simulink library "monroe_library"  (R2012b)
settings: Solver=ode45  StartTime=0.0  StopTime=10.0  RelTol=1e-3
values from neighbouring files (symbols this model uses):
  input_bit_width = ', num2str(input_bit_width))    [fft_direct_draw.m]
undefined symbols (not defined in the file or in its folder): gcbh, xlBlockLoadCallback
libraries: xbsIndex_r4 x1880, monroe_library x159, casper_library x13, xps_library x1
(part 5 of 43)

== system monroe_library/direct_coeff_gen ==
  sync : Inport
  bulk_delay_1 : Subsystem
  bulk_delay_2 : Subsystem
  bulk_delay_3 : Subsystem
  coeff_gen_stage_1_group_1 : Subsystem
  coeff_gen_stage_1_group_2 : Subsystem
  coeff_gen_stage_1_group_3 : Subsystem
  coeff_gen_stage_1_group_4 : Subsystem
  coeff_gen_stage_2_group_1 : Subsystem
  coeff_gen_stage_2_group_2 : Subsystem
  coeff_gen_stage_2_group_3 : Subsystem
  coeff_gen_stage_2_group_4 : Subsystem
  coeff_gen_stage_3_group_1 : Subsystem
  coeff_gen_stage_3_group_2 : Subsystem
  coeff_gen_stage_3_group_3 : Subsystem
  coeff_gen_stage_3_group_4 : Subsystem
  concat_stage_1 : xbsIndex_r4/Concat  num_inputs=4  dbl_ovrd=off  block_type=concat
  concat_stage_2 : xbsIndex_r4/Concat  num_inputs=4  dbl_ovrd=off  block_type=concat
  concat_stage_3 : xbsIndex_r4/Concat  num_inputs=4  dbl_ovrd=off  block_type=concat
  delay_sync_{1..2,4..5} (4 alike) : xbsIndex_r4/Delay  en=off  latency=1  dbl_ovrd=off  reg_retiming=off  block_type=delay
  delay_sync_3 : xbsIndex_r4/Delay  en=off  latency=36  dbl_ovrd=off  reg_retiming=off  block_type=delay
  coeff_stg1 : Outport
  coeff_stg2 : Outport  Port=2
  coeff_stg3 : Outport  Port=3
  sync_out : Outport  Port=4
  wires:
  sync/1 -> delay_sync_1/1, bulk_delay_1/4(in4), bulk_delay_1/3(in3), bulk_delay_1/2(in2), bulk_delay_1/1(in1)
  bulk_delay_1/1(out1) -> bulk_delay_2/1(in1), coeff_gen_stage_1_group_1/1(sync)
  bulk_delay_1/2(out2) -> bulk_delay_2/2(in2), coeff_gen_stage_1_group_2/1(sync)
  bulk_delay_1/3(out3) -> bulk_delay_2/3(in3), coeff_gen_stage_1_group_3/1(sync)
  bulk_delay_1/4(out4) -> bulk_delay_2/4(in4), coeff_gen_stage_1_group_4/1(sync)
  bulk_delay_2/1(out1) -> bulk_delay_3/1(in1), coeff_gen_stage_2_group_1/1(sync)
  bulk_delay_2/2(out2) -> bulk_delay_3/2(in2), coeff_gen_stage_2_group_2/1(sync)
  bulk_delay_2/3(out3) -> bulk_delay_3/3(in3), coeff_gen_stage_2_group_3/1(sync)
  bulk_delay_2/4(out4) -> bulk_delay_3/4(in4), coeff_gen_stage_2_group_4/1(sync)
  delay_sync_5/1 -> sync_out/1
  delay_sync_4/1 -> delay_sync_5/1
  delay_sync_3/1 -> delay_sync_4/1
  delay_sync_2/1 -> delay_sync_3/1
  delay_sync_1/1 -> delay_sync_2/1
  concat_stage_3/1 -> coeff_stg3/1
  coeff_gen_stage_3_group_4/1(coeff) -> concat_stage_3/4
  coeff_gen_stage_3_group_3/1(coeff) -> concat_stage_3/3
  coeff_gen_stage_3_group_2/1(coeff) -> concat_stage_3/2
  coeff_gen_stage_3_group_1/1(coeff) -> concat_stage_3/1
  bulk_delay_3/4(out4) -> coeff_gen_stage_3_group_4/1(sync)
  bulk_delay_3/3(out3) -> coeff_gen_stage_3_group_3/1(sync)
  bulk_delay_3/2(out2) -> coeff_gen_stage_3_group_2/1(sync)
  bulk_delay_3/1(out1) -> coeff_gen_stage_3_group_1/1(sync)
  concat_stage_2/1 -> coeff_stg2/1
  coeff_gen_stage_2_group_4/1(coeff) -> concat_stage_2/4
  coeff_gen_stage_2_group_3/1(coeff) -> concat_stage_2/3
  coeff_gen_stage_2_group_2/1(coeff) -> concat_stage_2/2
  coeff_gen_stage_2_group_1/1(coeff) -> concat_stage_2/1
  concat_stage_1/1 -> coeff_stg1/1
  coeff_gen_stage_1_group_4/1(coeff) -> concat_stage_1/4
  coeff_gen_stage_1_group_3/1(coeff) -> concat_stage_1/3
  coeff_gen_stage_1_group_2/1(coeff) -> concat_stage_1/2
  coeff_gen_stage_1_group_1/1(coeff) -> concat_stage_1/1

== system monroe_library/double_delay_bram_external_counter ==
  note: The delay length pramater is used to set the depth of the RAM.
  inA : Inport
  inB : Inport  Port=2
  count : Inport  Port=3
  Concat : xbsIndex_r4/Concat  num_inputs=2  dbl_ovrd=off  block_type=concat
  Concat1 : S-Function  LoadFcn=xlBlockLoadCallback(gcbh);  FunctionName=sysgen  Parameters=ptable_  EnableBusSupport=off  mask(Xilinx Bus Concatenator Block){infoedit=Concatenates two or more inputs.  Output will be cast to an unsigned value with the binary point at zero., num_inputs=2, dbl_ovrd_sgadvanced=, dbl_ovrd=off, has_advanced_control=0, sggui_pos=-1,-1,-1,-1, block_type=concat, block_version=, sg_icon_stat=60,60,2,1,white,blue,0,16398980,right,,[ ],[ ], sg_mask_display=|, sg_list_contents=, sg_blockgui_xml=}
      mask sg_mask_display=|
      | fprintf('','COMMENT: begin icon graphics');
      | patch([0 60 60 0 0 ],[0 0 60 60 0 ],[0.77 0.82 0.91 ]);
      | plot([0 60 60 0 0 ],[0 0 60 60 0 ]);
      | patch([12.2 23.76 31.76 39.76 47.76 31.76 20.2 12.2 ],[38.88 38.88 46.88 38.88 46.88 46.88 46.88 38.88 ],[1 1 1 ]);
      | patch([20.2 31.76 23.76 12.2 20.2 ],[30.88 30.88 38.88 38.88 30.88 ],[0.931 0.946 0.973 ]);
      | patch([12.2 23.76 31.76 20.2 12.2 ],[22.88 22.88 30.88 30.88 22.88 ],[1 1 1 ]);
      | patch([20.2 47.76 39.76 31.76 23.76 12.2 20.2 ],[14.88 14.88 22.88 14.88 22.88 22.88 14.88 ],[0.931 0.946 0.973 ]);
      | fprintf('','COMMENT: end icon graphics');
      | fprintf('','COMMENT: begin icon text');
      | color('black');port_label('input',1,'hi');
      | color('black');port_label('input',2,'lo');
      |
      | color('black');disp('\fontsize{20}\}','texmode','on');
      | fprintf('','COMMENT: end icon text');
      mask prompts: infoedit ""; num_inputs "Number of inputs"; dbl_ovrd_sgadvanced ""; dbl_ovrd "Override with doubles"; has_advanced_control ""; sggui_pos ""; block_type ""; block_version ""; sg_icon_stat ""; sg_mask_display ""; sg_list_contents ""; sg_blockgui_xml ""
      mask help: Concatenates two or more inputs. Output will be cast to an unsigned value with the binary point at zero.
      mask init:
      | try
      |   tmp_gcb = gcb;
      |   tmp_gcbh = gcbh;
      |   if (strcmp('SysGenIndex',get_param(bdroot(tmp_gcbh),'tag')) && ~isempty(regexp(bdroot(tmp_gcb), '^xbs', 'once')))
      |     return;
      |   end;
      |   xlMungeMaskParams;
      |   block_config = 'sysgen_blockset:Concat_config';
      | 
      |   block_type='concat';
      | 
      |   serialized_declarations = '{''num_inputs''=>''Int'',''sim_engine''=>''Int'',''sysgen_root''=>''String'',''block_type''=>''String''}';
      |   xlconcat_init();
      |   ptable_ = xlblockprep(get_param(tmp_gcb, 'MaskWSVariables'));
      |   try
      |     xlBlockMoveCallback(tmp_gcbh);
      |   catch 
      |      clear global xl_updateicon_recursion_guard;
      |   end;
      | catch
      |   global dbgsysgen;
      |   if(~isempty(dbgsysgen) && dbgsysgen)
      |     e = regexprep(lasterr, '\n', '\nError: ');
      |     disp(['Error: While running MaskInit code on block ' tmp_gcb ': ' e]);
      |     error(e);
      |   end
      | end
      settings: CopyFcn=xlBlockMoveCallback(gcbh);  DeleteFcn=xlDestroyGui(gcbh);  ModelCloseFcn=xlDestroyGui(gcbh);  PreSaveFcn=xlBlockPreSaveCallback(gcbh);  PostSaveFcn=xlBlockPostSaveCallback(gcbh);  DestroyFcn=xlDestroyGui(gcbh);  OpenFcn=xlOpenGui(gcbh, 'concat_gui.xml', @xlmagicenablement, -1)  CloseFcn=xlDestroyGui(gcbh);  MoveFcn=xlBlockMoveCallback(gcbh);
      mask Help: eval('');xlDoc('-book','sysgen','-topic','Concat');
      mask Display:
      | fprintf('','COMMENT: begin icon graphics');
      | patch([0 60 60 0 0 ],[0 0 60 60 0 ],[0.77 0.82 0.91 ]);
      | plot([0 60 60 0 0 ],[0 0 60 60 0 ]);
      | patch([12.2 23.76 31.76 39.76 47.76 31.76 20.2 12.2 ],[38.88 38.88 46.88 38.88 46.88 46.88 46.88 38.88 ],[1 1 1 ]);
      | patch([20.2 31.76 23.76 12.2 20.2 ],[30.88 30.88 38.88 38.88 30.88 ],[0.931 0.946 0.973 ]);
      | patch([12.2 23.76 31.76 20.2 12.2 ],[22.88 22.88 30.88 30.88 22.88 ],[1 1 1 ]);
      | patch([20.2 47.76 39.76 31.76 23.76 12.2 20.2 ],[14.88 14.88 22.88 14.88 22.88 22.88 14.88 ],[0.931 0.946 0.973 ]);
      | fprintf('','COMMENT: end icon graphics');
      | fprintf('','COMMENT: begin icon text');
      | color('black');port_label('input',1,'hi');
      | color('black');port_label('input',2,'lo');
      | 
      | color('black');disp('\fontsize{20}\}','texmode','on');
      | fprintf('','COMMENT: end icon text');
  Constant1 : xbsIndex_r4/Constant  arith_type=Boolean  const=1  n_bits=1  bin_pt=0  explicit_period=on  period=1  equ=P=C  opselect=C  inp2=PCIN>>17  opr=+  inp1=P  carry=CIN  dbl_ovrd=off  block_type=constant
      settings: block_version=9.1.01
  Constant2 : xbsIndex_r4/Constant  arith_type=Boolean  const=1  n_bits=1  bin_pt=0  explicit_period=on  period=1  equ=P=C  opselect=C  inp2=PCIN>>17  opr=+  inp1=P  carry=CIN  dbl_ovrd=off  block_type=constant
      settings: block_version=9.1.01
  Constant3 : S-Function  LoadFcn=xlBlockLoadCallback(gcbh);  FunctionName=sysgen  Parameters=ptable_  EnableBusSupport=off  mask(Xilinx Constant Block Block){arith_type_sgadvanced=, arith_type=Boolean, const=0, n_bits=1, bin_pt=0, explicit_period_sgadvanced=, explicit_period=on, period=1, dsp48_infoedit=The use of this block for DSP48 instructions is deprecated.  Please use the Opmode block., equ=P=C, opselect_sgadvanced=, opselect=C, inp2_sgadvanced=, inp2=PCIN>>17, opr_sgadvanced=, opr=+, inp1_sgadvanced=, inp1=P, carry_sgadvanced=, carry=CIN, dbl_ovrd_sgadvanced=, dbl_ovrd=off, has_advanced_control=0, sggui_pos=-1,-1,-1,-1, block_type=constant, block_version=9.1.01, sg_icon_stat=35,24,0,1,white,blue,0,bf4ddd8b,right,,[ ],[ ], sg_mask_display=|, sg_list_contents=, sg_blockgui_xml=}
      mask sg_mask_display=|
      | fprintf('','COMMENT: begin icon graphics');
      | patch([0 35 35 0 0 ],[0 0 24 24 0 ],[0.77 0.82 0.91 ]);
      | plot([0 35 35 0 0 ],[0 0 24 24 0 ]);
      | patch([10.325 14.66 17.66 20.66 23.66 17.66 13.325 10.325 ],[15.33 15.33 18.33 15.33 18.33 18.33 18.33 15.33 ],[1 1 1 ]);
      | patch([13.325 17.66 14.66 10.325 13.325 ],[12.33 12.33 15.33 15.33 12.33 ],[0.931 0.946 0.973 ]);
      | patch([10.325 14.66 17.66 13.325 10.325 ],[9.33 9.33 12.33 12.33 9.33 ],[1 1 1 ]);
      | patch([13.325 23.66 20.66 17.66 14.66 10.325 13.325 ],[6.33 6.33 9.33 6.33 9.33 9.33 6.33 ],[0.931 0.946 0.973 ]);
      | fprintf('','COMMENT: end icon graphics');
      | fprintf('','COMMENT: begin icon text');
      | color('black');port_label('output',1,'0');
      | fprintf('','COMMENT: end icon text');
      mask prompts: arith_type_sgadvanced ""; arith_type "Type"; const "Constant value"; n_bits "Number of bits"; bin_pt "Binary point"; explicit_period_sgadvanced ""; explicit_period "Sampled constant"; period "Sample period"; dsp48_infoedit ""; equ "DSP48 operation"; opselect_sgadvanced ""; opselect "Operation select"; inp2_sgadvanced ""; inp2 "Z mux"; opr_sgadvanced ""; opr "Operand"; inp1_sgadvanced ""; inp1 "YX muxes"; carry_sgadvanced ""; carry "Carry input"; dbl_ovrd_sgadvanced ""; dbl_ovrd "Override with doubles"; has_advanced_control ""; sggui_pos ""; block_type ""; block_version ""; sg_icon_stat ""; sg_mask_display ""; sg_list_contents ""; sg_blockgui_xml ""
      mask help: Xilinx Constant Block
      mask init:
      | try
      |   tmp_gcb = gcb;
      |   tmp_gcbh = gcbh;
      |   if (strcmp('SysGenIndex',get_param(bdroot(tmp_gcbh),'tag')) && ~isempty(regexp(bdroot(tmp_gcb), '^xbs', 'once')))
      |     return;
      |   end;
      |   xlMungeMaskParams;
      |   block_config = 'sysgen_blockset:Constant_config';
      | 
      |   block_type='constant';
      | 
      |   serialized_declarations = '{''arith_type''=>''Int'',''bin_pt''=>''Int'',''carry''=>''Int'',''const''=>''Double'',''dbl_ovrd''=>''Int'',''explicit_period''=>''Int'',''inp1''=>''Int'',''inp2''=>''Int'',''n_bits''=>''Int'',''opr''=>''Int'',''opselect''=>''Int'',''period''=>''Double'',''block_type''=>''String''}';
      |   xlconstant_init();
      |   ptable_ = xlblockprep(get_param(tmp_gcb, 'MaskWSVariables'));
      |   try
      |     xlBlockMoveCallback(tmp_gcbh);
      |   catch 
      |      clear global xl_updateicon_recursion_guard;
      |   end;
      | catch
      |   global dbgsysgen;
      |   if(~isempty(dbgsysgen) && dbgsysgen)
      |     e = regexprep(lasterr, '\n', '\nError: ');
      |     disp(['Error: While running MaskInit code on block ' tmp_gcb ': ' e]);
      |     error(e);
      |   end
      | end
      settings: CopyFcn=xlBlockMoveCallback(gcbh);  DeleteFcn=xlDestroyGui(gcbh);  ModelCloseFcn=xlDestroyGui(gcbh);  PreSaveFcn=xlBlockPreSaveCallback(gcbh);  PostSaveFcn=xlBlockPostSaveCallback(gcbh);  DestroyFcn=xlDestroyGui(gcbh);  OpenFcn=xlOpenGui(gcbh, 'constant_gui.xml', @constantenablement, @constantaction)  CloseFcn=xlDestroyGui(gcbh);  MoveFcn=xlBlockMoveCallback(gcbh);
      mask Help: eval('');xlDoc('-book','sysgen','-topic','Constant');
      mask TypeOptions arith_type: Boolean | Signed (2's comp) | Unsigned | DSP48 Instruction
      mask TypeOptions opselect: C + A*B | PCIN + A*B | P + A*B | A * B | C + A:B | C - A:B | C | Custom
      mask TypeOptions inp2: 0 | PCIN | P | C | PCIN>>17 | P>>17
      mask TypeOptions opr: + | -
      mask TypeOptions inp1: 0 | P | A:B | A*B | C | P+C | A:B+C
      mask TypeOptions carry: 0 | 1 | CIN | ~SIGN(P or PCIN) | ~SIGN(A*B or A:B) | ~SIGND(A*B or A:B)
      mask Display:
      | fprintf('','COMMENT: begin icon graphics');
      | patch([0 35 35 0 0 ],[0 0 24 24 0 ],[0.77 0.82 0.91 ]);
      | plot([0 35 35 0 0 ],[0 0 24 24 0 ]);
      | patch([10.325 14.66 17.66 20.66 23.66 17.66 13.325 10.325 ],[15.33 15.33 18.33 15.33 18.33 18.33 18.33 15.33 ],[1 1 1 ]);
      | patch([13.325 17.66 14.66 10.325 13.325 ],[12.33 12.33 15.33 15.33 12.33 ],[0.931 0.946 0.973 ]);
      | patch([10.325 14.66 17.66 13.325 10.325 ],[9.33 9.33 12.33 12.33 9.33 ],[1 1 1 ]);
      | patch([13.325 23.66 20.66 17.66 14.66 10.325 13.325 ],[6.33 6.33 9.33 6.33 9.33 9.33 6.33 ],[0.931 0.946 0.973 ]);
      | fprintf('','COMMENT: end icon graphics');
      | fprintf('','COMMENT: begin icon text');
      | color('black');port_label('output',1,'0');
      | fprintf('','COMMENT: end icon text');
  Dual Port RAM : xbsIndex_r4/Dual Port RAM  depth=2^ceil(log(2*(delay_len-bram_latency))/log(2))  initVector=0  distributed_mem=Block RAM  init_a=0  init_b=0  rst_a=off  rst_b=off  en_a=off  en_b=off  latency=bram_latency  write_mode_A=Read Before Write  write_mode_B=Read Before Write  dbl_ovrd=off  optimize=Area  use_rpm=on  block_type=dpram
      settings: block_version=11.4
  outA : Outport
  outB : Outport  Port=2
  wires:
  Constant3/1 -> Concat1/1
  Concat1/1 -> Dual Port RAM/4
  Concat/1 -> Dual Port RAM/1
  Constant1/1 -> Concat/1
  count/1 -> Concat1/2, Concat/2
  Constant2/1 -> Dual Port RAM/3, Dual Port RAM/6
  inB/1 -> Dual Port RAM/5
  inA/1 -> Dual Port RAM/2
  Dual Port RAM/2 -> outB/1
  Dual Port RAM/1 -> outA/1

== system monroe_library/double_delay_bram_fast ==
  inA : Inport
  inB : Inport  Port=2
  Concat : xbsIndex_r4/Concat  num_inputs=2  dbl_ovrd=off  block_type=concat
  Concat1 : S-Function  LoadFcn=xlBlockLoadCallback(gcbh);  FunctionName=sysgen  Parameters=ptable_  EnableBusSupport=off  mask(Xilinx Bus Concatenator Block){infoedit=Concatenates two or more inputs.  Output will be cast to an unsigned value with the binary point at zero., num_inputs=2, dbl_ovrd_sgadvanced=, dbl_ovrd=off, has_advanced_control=0, sggui_pos=-1,-1,-1,-1, block_type=concat, block_version=, sg_icon_stat=60,60,2,1,white,blue,0,16398980,right,,[ ],[ ], sg_mask_display=|, sg_list_contents=, sg_blockgui_xml=}
      mask sg_mask_display=|
      | fprintf('','COMMENT: begin icon graphics');
      | patch([0 60 60 0 0 ],[0 0 60 60 0 ],[0.77 0.82 0.91 ]);
      | plot([0 60 60 0 0 ],[0 0 60 60 0 ]);
      | patch([12.2 23.76 31.76 39.76 47.76 31.76 20.2 12.2 ],[38.88 38.88 46.88 38.88 46.88 46.88 46.88 38.88 ],[1 1 1 ]);
      | patch([20.2 31.76 23.76 12.2 20.2 ],[30.88 30.88 38.88 38.88 30.88 ],[0.931 0.946 0.973 ]);
      | patch([12.2 23.76 31.76 20.2 12.2 ],[22.88 22.88 30.88 30.88 22.88 ],[1 1 1 ]);
      | patch([20.2 47.76 39.76 31.76 23.76 12.2 20.2 ],[14.88 14.88 22.88 14.88 22.88 22.88 14.88 ],[0.931 0.946 0.973 ]);
      | fprintf('','COMMENT: end icon graphics');
      | fprintf('','COMMENT: begin icon text');
      | color('black');port_label('input',1,'hi');
      | color('black');port_label('input',2,'lo');
      |
      | color('black');disp('\fontsize{20}\}','texmode','on');
      | fprintf('','COMMENT: end icon text');
      mask prompts: infoedit ""; num_inputs "Number of inputs"; dbl_ovrd_sgadvanced ""; dbl_ovrd "Override with doubles"; has_advanced_control ""; sggui_pos ""; block_type ""; block_version ""; sg_icon_stat ""; sg_mask_display ""; sg_list_contents ""; sg_blockgui_xml ""
      mask help: Concatenates two or more inputs. Output will be cast to an unsigned value with the binary point at zero.
      mask init: same as monroe_library/double_delay_bram_external_counter/Concat1
      settings: CopyFcn=xlBlockMoveCallback(gcbh);  DeleteFcn=xlDestroyGui(gcbh);  ModelCloseFcn=xlDestroyGui(gcbh);  PreSaveFcn=xlBlockPreSaveCallback(gcbh);  PostSaveFcn=xlBlockPostSaveCallback(gcbh);  DestroyFcn=xlDestroyGui(gcbh);  OpenFcn=xlOpenGui(gcbh, 'concat_gui.xml', @xlmagicenablement, -1)  CloseFcn=xlDestroyGui(gcbh);  MoveFcn=xlBlockMoveCallback(gcbh);
      mask Help: eval('');xlDoc('-book','sysgen','-topic','Concat');
      mask Display:
      | fprintf('','COMMENT: begin icon graphics');
      | patch([0 60 60 0 0 ],[0 0 60 60 0 ],[0.77 0.82 0.91 ]);
      | plot([0 60 60 0 0 ],[0 0 60 60 0 ]);
      | patch([12.2 23.76 31.76 39.76 47.76 31.76 20.2 12.2 ],[38.88 38.88 46.88 38.88 46.88 46.88 46.88 38.88 ],[1 1 1 ]);
      | patch([20.2 31.76 23.76 12.2 20.2 ],[30.88 30.88 38.88 38.88 30.88 ],[0.931 0.946 0.973 ]);
      | patch([12.2 23.76 31.76 20.2 12.2 ],[22.88 22.88 30.88 30.88 22.88 ],[1 1 1 ]);
      | patch([20.2 47.76 39.76 31.76 23.76 12.2 20.2 ],[14.88 14.88 22.88 14.88 22.88 22.88 14.88 ],[0.931 0.946 0.973 ]);
      | fprintf('','COMMENT: end icon graphics');
      | fprintf('','COMMENT: begin icon text');
      | color('black');port_label('input',1,'hi');
      | color('black');port_label('input',2,'lo');
      | 
      | color('black');disp('\fontsize{20}\}','texmode','on');
      | fprintf('','COMMENT: end icon text');
  Constant1 : xbsIndex_r4/Constant  arith_type=Boolean  const=1  n_bits=1  bin_pt=0  explicit_period=on  period=1  equ=P=C  opselect=C  inp2=PCIN>>17  opr=+  inp1=P  carry=CIN  dbl_ovrd=off  block_type=constant
      settings: block_version=9.1.01
  Constant2 : xbsIndex_r4/Constant  arith_type=Boolean  const=1  n_bits=1  bin_pt=0  explicit_period=on  period=1  equ=P=C  opselect=C  inp2=PCIN>>17  opr=+  inp1=P  carry=CIN  dbl_ovrd=off  block_type=constant
      settings: block_version=9.1.01
  Constant3 : S-Function  LoadFcn=xlBlockLoadCallback(gcbh);  FunctionName=sysgen  Parameters=ptable_  EnableBusSupport=off  mask(Xilinx Constant Block Block){arith_type_sgadvanced=, arith_type=Boolean, const=0, n_bits=1, bin_pt=0, explicit_period_sgadvanced=, explicit_period=on, period=1, dsp48_infoedit=The use of this block for DSP48 instructions is deprecated.  Please use the Opmode block., equ=P=C, opselect_sgadvanced=, opselect=C, inp2_sgadvanced=, inp2=PCIN>>17, opr_sgadvanced=, opr=+, inp1_sgadvanced=, inp1=P, carry_sgadvanced=, carry=CIN, dbl_ovrd_sgadvanced=, dbl_ovrd=off, has_advanced_control=0, sggui_pos=-1,-1,-1,-1, block_type=constant, block_version=9.1.01, sg_icon_stat=35,24,0,1,white,blue,0,bf4ddd8b,right,,[ ],[ ], sg_mask_display=|, sg_list_contents=, sg_blockgui_xml=}
      mask sg_mask_display=|
      | fprintf('','COMMENT: begin icon graphics');
      | patch([0 35 35 0 0 ],[0 0 24 24 0 ],[0.77 0.82 0.91 ]);
      | plot([0 35 35 0 0 ],[0 0 24 24 0 ]);
      | patch([10.325 14.66 17.66 20.66 23.66 17.66 13.325 10.325 ],[15.33 15.33 18.33 15.33 18.33 18.33 18.33 15.33 ],[1 1 1 ]);
      | patch([13.325 17.66 14.66 10.325 13.325 ],[12.33 12.33 15.33 15.33 12.33 ],[0.931 0.946 0.973 ]);
      | patch([10.325 14.66 17.66 13.325 10.325 ],[9.33 9.33 12.33 12.33 9.33 ],[1 1 1 ]);
      | patch([13.325 23.66 20.66 17.66 14.66 10.325 13.325 ],[6.33 6.33 9.33 6.33 9.33 9.33 6.33 ],[0.931 0.946 0.973 ]);
      | fprintf('','COMMENT: end icon graphics');
      | fprintf('','COMMENT: begin icon text');
      | color('black');port_label('output',1,'0');
      | fprintf('','COMMENT: end icon text');
      mask prompts: arith_type_sgadvanced ""; arith_type "Type"; const "Constant value"; n_bits "Number of bits"; bin_pt "Binary point"; explicit_period_sgadvanced ""; explicit_period "Sampled constant"; period "Sample period"; dsp48_infoedit ""; equ "DSP48 operation"; opselect_sgadvanced ""; opselect "Operation select"; inp2_sgadvanced ""; inp2 "Z mux"; opr_sgadvanced ""; opr "Operand"; inp1_sgadvanced ""; inp1 "YX muxes"; carry_sgadvanced ""; carry "Carry input"; dbl_ovrd_sgadvanced ""; dbl_ovrd "Override with doubles"; has_advanced_control ""; sggui_pos ""; block_type ""; block_version ""; sg_icon_stat ""; sg_mask_display ""; sg_list_contents ""; sg_blockgui_xml ""
      mask help: Xilinx Constant Block
      mask init: same as monroe_library/double_delay_bram_external_counter/Constant3
      settings: CopyFcn=xlBlockMoveCallback(gcbh);  DeleteFcn=xlDestroyGui(gcbh);  ModelCloseFcn=xlDestroyGui(gcbh);  PreSaveFcn=xlBlockPreSaveCallback(gcbh);  PostSaveFcn=xlBlockPostSaveCallback(gcbh);  DestroyFcn=xlDestroyGui(gcbh);  OpenFcn=xlOpenGui(gcbh, 'constant_gui.xml', @constantenablement, @constantaction)  CloseFcn=xlDestroyGui(gcbh);  MoveFcn=xlBlockMoveCallback(gcbh);
      mask Help: eval('');xlDoc('-book','sysgen','-topic','Constant');
      mask TypeOptions arith_type: Boolean | Signed (2's comp) | Unsigned | DSP48 Instruction
      mask TypeOptions opselect: C + A*B | PCIN + A*B | P + A*B | A * B | C + A:B | C - A:B | C | Custom
      mask TypeOptions inp2: 0 | PCIN | P | C | PCIN>>17 | P>>17
      mask TypeOptions opr: + | -
      mask TypeOptions inp1: 0 | P | A:B | A*B | C | P+C | A:B+C
      mask TypeOptions carry: 0 | 1 | CIN | ~SIGN(P or PCIN) | ~SIGN(A*B or A:B) | ~SIGND(A*B or A:B)
      mask Display:
      | fprintf('','COMMENT: begin icon graphics');
      | patch([0 35 35 0 0 ],[0 0 24 24 0 ],[0.77 0.82 0.91 ]);
      | plot([0 35 35 0 0 ],[0 0 24 24 0 ]);
      | patch([10.325 14.66 17.66 20.66 23.66 17.66 13.325 10.325 ],[15.33 15.33 18.33 15.33 18.33 18.33 18.33 15.33 ],[1 1 1 ]);
      | patch([13.325 17.66 14.66 10.325 13.325 ],[12.33 12.33 15.33 15.33 12.33 ],[0.931 0.946 0.973 ]);
      | patch([10.325 14.66 17.66 13.325 10.325 ],[9.33 9.33 12.33 12.33 9.33 ],[1 1 1 ]);
      | patch([13.325 23.66 20.66 17.66 14.66 10.325 13.325 ],[6.33 6.33 9.33 6.33 9.33 9.33 6.33 ],[0.931 0.946 0.973 ]);
      | fprintf('','COMMENT: end icon graphics');
      | fprintf('','COMMENT: begin icon text');
      | color('black');port_label('output',1,'0');
      | fprintf('','COMMENT: end icon text');
  Dual Port RAM : xbsIndex_r4/Dual Port RAM  depth=2^ceil(log(2*(delay_len-bram_latency))/log(2))  initVector=0  distributed_mem=Block RAM  init_a=0  init_b=0  rst_a=off  rst_b=off  en_a=off  en_b=off  latency=bram_latency  write_mode_A=Read Before Write  write_mode_B=Read Before Write  dbl_ovrd=off  optimize=Area  use_rpm=on  block_type=dpram
      settings: block_version=11.4
  counter_limited_fast : monroe_library/counter_limited_fast  SystemSampleTime=-1  bit_width=ceil(log(delay_len-bram_latency)/log(2))  count_to=delay_len-bram_latency-1  register_output=register_counter  cheap_counter=((ceil(log(delay_len-bram_latency)/log(2))) < 8)
  outA : Outport
  outB : Outport  Port=2
  wires:
  Dual Port RAM/1 -> outA/1
  Dual Port RAM/2 -> outB/1
  inA/1 -> Dual Port RAM/2
  inB/1 -> Dual Port RAM/5
  Constant2/1 -> Dual Port RAM/6, Dual Port RAM/3
  counter_limited_fast/1 -> Concat/2, Concat1/2
  Constant1/1 -> Concat/1
  Concat/1 -> Dual Port RAM/1
  Concat1/1 -> Dual Port RAM/4
  Constant3/1 -> Concat1/1

== system monroe_library/double_delay_distrib ==
  inA : Inport
  inB : Inport  Port=2
  Concat : xbsIndex_r4/Concat  num_inputs=2  dbl_ovrd=off  block_type=concat
  Concat1 : S-Function  LoadFcn=xlBlockLoadCallback(gcbh);  FunctionName=sysgen  Parameters=ptable_  EnableBusSupport=off  mask(Xilinx Bus Concatenator Block){infoedit=Concatenates two or more inputs.  Output will be cast to an unsigned value with the binary point at zero., num_inputs=2, dbl_ovrd_sgadvanced=, dbl_ovrd=off, has_advanced_control=0, sggui_pos=-1,-1,-1,-1, block_type=concat, block_version=, sg_icon_stat=60,60,2,1,white,blue,0,16398980,right,,[ ],[ ], sg_mask_display=|, sg_list_contents=, sg_blockgui_xml=}
      mask sg_mask_display=|
      | fprintf('','COMMENT: begin icon graphics');
      | patch([0 60 60 0 0 ],[0 0 60 60 0 ],[0.77 0.82 0.91 ]);
      | plot([0 60 60 0 0 ],[0 0 60 60 0 ]);
      | patch([12.2 23.76 31.76 39.76 47.76 31.76 20.2 12.2 ],[38.88 38.88 46.88 38.88 46.88 46.88 46.88 38.88 ],[1 1 1 ]);
      | patch([20.2 31.76 23.76 12.2 20.2 ],[30.88 30.88 38.88 38.88 30.88 ],[0.931 0.946 0.973 ]);
      | patch([12.2 23.76 31.76 20.2 12.2 ],[22.88 22.88 30.88 30.88 22.88 ],[1 1 1 ]);
      | patch([20.2 47.76 39.76 31.76 23.76 12.2 20.2 ],[14.88 14.88 22.88 14.88 22.88 22.88 14.88 ],[0.931 0.946 0.973 ]);
      | fprintf('','COMMENT: end icon graphics');
      | fprintf('','COMMENT: begin icon text');
      | color('black');port_label('input',1,'hi');
      | color('black');port_label('input',2,'lo');
      |
      | color('black');disp('\fontsize{20}\}','texmode','on');
      | fprintf('','COMMENT: end icon text');
      mask prompts: infoedit ""; num_inputs "Number of inputs"; dbl_ovrd_sgadvanced ""; dbl_ovrd "Override with doubles"; has_advanced_control ""; sggui_pos ""; block_type ""; block_version ""; sg_icon_stat ""; sg_mask_display ""; sg_list_contents ""; sg_blockgui_xml ""
      mask help: Concatenates two or more inputs. Output will be cast to an unsigned value with the binary point at zero.
      mask init: same as monroe_library/double_delay_bram_external_counter/Concat1
      settings: CopyFcn=xlBlockMoveCallback(gcbh);  DeleteFcn=xlDestroyGui(gcbh);  ModelCloseFcn=xlDestroyGui(gcbh);  PreSaveFcn=xlBlockPreSaveCallback(gcbh);  PostSaveFcn=xlBlockPostSaveCallback(gcbh);  DestroyFcn=xlDestroyGui(gcbh);  OpenFcn=xlOpenGui(gcbh, 'concat_gui.xml', @xlmagicenablement, -1)  CloseFcn=xlDestroyGui(gcbh);  MoveFcn=xlBlockMoveCallback(gcbh);
      mask Help: eval('');xlDoc('-book','sysgen','-topic','Concat');
      mask Display:
      | fprintf('','COMMENT: begin icon graphics');
      | patch([0 60 60 0 0 ],[0 0 60 60 0 ],[0.77 0.82 0.91 ]);
      | plot([0 60 60 0 0 ],[0 0 60 60 0 ]);
      | patch([12.2 23.76 31.76 39.76 47.76 31.76 20.2 12.2 ],[38.88 38.88 46.88 38.88 46.88 46.88 46.88 38.88 ],[1 1 1 ]);
      | patch([20.2 31.76 23.76 12.2 20.2 ],[30.88 30.88 38.88 38.88 30.88 ],[0.931 0.946 0.973 ]);
      | patch([12.2 23.76 31.76 20.2 12.2 ],[22.88 22.88 30.88 30.88 22.88 ],[1 1 1 ]);
      | patch([20.2 47.76 39.76 31.76 23.76 12.2 20.2 ],[14.88 14.88 22.88 14.88 22.88 22.88 14.88 ],[0.931 0.946 0.973 ]);
      | fprintf('','COMMENT: end icon graphics');
      | fprintf('','COMMENT: begin icon text');
      | color('black');port_label('input',1,'hi');
      | color('black');port_label('input',2,'lo');
      | 
      | color('black');disp('\fontsize{20}\}','texmode','on');
      | fprintf('','COMMENT: end icon text');
  Constant1 : xbsIndex_r4/Constant  arith_type=Boolean  const=1  n_bits=1  bin_pt=0  explicit_period=on  period=1  equ=P=C  opselect=C  inp2=PCIN>>17  opr=+  inp1=P  carry=CIN  dbl_ovrd=off  block_type=constant
      settings: block_version=9.1.01
  Constant2 : xbsIndex_r4/Constant  arith_type=Boolean  const=1  n_bits=1  bin_pt=0  explicit_period=on  period=1  equ=P=C  opselect=C  inp2=PCIN>>17  opr=+  inp1=P  carry=CIN  dbl_ovrd=off  block_type=constant
      settings: block_version=9.1.01
  Constant3 : S-Function  LoadFcn=xlBlockLoadCallback(gcbh);  FunctionName=sysgen  Parameters=ptable_  EnableBusSupport=off  mask(Xilinx Constant Block Block){arith_type_sgadvanced=, arith_type=Boolean, const=0, n_bits=1, bin_pt=0, explicit_period_sgadvanced=, explicit_period=on, period=1, dsp48_infoedit=The use of this block for DSP48 instructions is deprecated.  Please use the Opmode block., equ=P=C, opselect_sgadvanced=, opselect=C, inp2_sgadvanced=, inp2=PCIN>>17, opr_sgadvanced=, opr=+, inp1_sgadvanced=, inp1=P, carry_sgadvanced=, carry=CIN, dbl_ovrd_sgadvanced=, dbl_ovrd=off, has_advanced_control=0, sggui_pos=-1,-1,-1,-1, block_type=constant, block_version=9.1.01, sg_icon_stat=35,24,0,1,white,blue,0,bf4ddd8b,right,,[ ],[ ], sg_mask_display=|, sg_list_contents=, sg_blockgui_xml=}
      mask sg_mask_display=|
      | fprintf('','COMMENT: begin icon graphics');
      | patch([0 35 35 0 0 ],[0 0 24 24 0 ],[0.77 0.82 0.91 ]);
      | plot([0 35 35 0 0 ],[0 0 24 24 0 ]);
      | patch([10.325 14.66 17.66 20.66 23.66 17.66 13.325 10.325 ],[15.33 15.33 18.33 15.33 18.33 18.33 18.33 15.33 ],[1 1 1 ]);
      | patch([13.325 17.66 14.66 10.325 13.325 ],[12.33 12.33 15.33 15.33 12.33 ],[0.931 0.946 0.973 ]);
      | patch([10.325 14.66 17.66 13.325 10.325 ],[9.33 9.33 12.33 12.33 9.33 ],[1 1 1 ]);
      | patch([13.325 23.66 20.66 17.66 14.66 10.325 13.325 ],[6.33 6.33 9.33 6.33 9.33 9.33 6.33 ],[0.931 0.946 0.973 ]);
      | fprintf('','COMMENT: end icon graphics');
      | fprintf('','COMMENT: begin icon text');
      | color('black');port_label('output',1,'0');
      | fprintf('','COMMENT: end icon text');
      mask prompts: arith_type_sgadvanced ""; arith_type "Type"; const "Constant value"; n_bits "Number of bits"; bin_pt "Binary point"; explicit_period_sgadvanced ""; explicit_period "Sampled constant"; period "Sample period"; dsp48_infoedit ""; equ "DSP48 operation"; opselect_sgadvanced ""; opselect "Operation select"; inp2_sgadvanced ""; inp2 "Z mux"; opr_sgadvanced ""; opr "Operand"; inp1_sgadvanced ""; inp1 "YX muxes"; carry_sgadvanced ""; carry "Carry input"; dbl_ovrd_sgadvanced ""; dbl_ovrd "Override with doubles"; has_advanced_control ""; sggui_pos ""; block_type ""; block_version ""; sg_icon_stat ""; sg_mask_display ""; sg_list_contents ""; sg_blockgui_xml ""
      mask help: Xilinx Constant Block
      mask init: same as monroe_library/double_delay_bram_external_counter/Constant3
      settings: CopyFcn=xlBlockMoveCallback(gcbh);  DeleteFcn=xlDestroyGui(gcbh);  ModelCloseFcn=xlDestroyGui(gcbh);  PreSaveFcn=xlBlockPreSaveCallback(gcbh);  PostSaveFcn=xlBlockPostSaveCallback(gcbh);  DestroyFcn=xlDestroyGui(gcbh);  OpenFcn=xlOpenGui(gcbh, 'constant_gui.xml', @constantenablement, @constantaction)  CloseFcn=xlDestroyGui(gcbh);  MoveFcn=xlBlockMoveCallback(gcbh);
      mask Help: eval('');xlDoc('-book','sysgen','-topic','Constant');
      mask TypeOptions arith_type: Boolean | Signed (2's comp) | Unsigned | DSP48 Instruction
      mask TypeOptions opselect: C + A*B | PCIN + A*B | P + A*B | A * B | C + A:B | C - A:B | C | Custom
      mask TypeOptions inp2: 0 | PCIN | P | C | PCIN>>17 | P>>17
      mask TypeOptions opr: + | -
      mask TypeOptions inp1: 0 | P | A:B | A*B | C | P+C | A:B+C
      mask TypeOptions carry: 0 | 1 | CIN | ~SIGN(P or PCIN) | ~SIGN(A*B or A:B) | ~SIGND(A*B or A:B)
      mask Display:
      | fprintf('','COMMENT: begin icon graphics');
      | patch([0 35 35 0 0 ],[0 0 24 24 0 ],[0.77 0.82 0.91 ]);
      | plot([0 35 35 0 0 ],[0 0 24 24 0 ]);
      | patch([10.325 14.66 17.66 20.66 23.66 17.66 13.325 10.325 ],[15.33 15.33 18.33 15.33 18.33 18.33 18.33 15.33 ],[1 1 1 ]);
      | patch([13.325 17.66 14.66 10.325 13.325 ],[12.33 12.33 15.33 15.33 12.33 ],[0.931 0.946 0.973 ]);
      | patch([10.325 14.66 17.66 13.325 10.325 ],[9.33 9.33 12.33 12.33 9.33 ],[1 1 1 ]);
      | patch([13.325 23.66 20.66 17.66 14.66 10.325 13.325 ],[6.33 6.33 9.33 6.33 9.33 9.33 6.33 ],[0.931 0.946 0.973 ]);
      | fprintf('','COMMENT: end icon graphics');
      | fprintf('','COMMENT: begin icon text');
      | color('black');port_label('output',1,'0');
      | fprintf('','COMMENT: end icon text');
  Counter : S-Function  LoadFcn=xlBlockLoadCallback(gcbh);  FunctionName=sysgen  Parameters=ptable_  EnableBusSupport=off  mask(Xilinx Counter Block){infoedit=Hardware notes: Free running counters are the least expensive in hardware.  A count limited counter is implemented by combining a counter with a comparator., cnt_type_sgadvanced=, cnt_type=Count Limited, cnt_to=delay_len-bram_latency-1, operation_sgadvanced=, operation=Up, start_count=0, cnt_by_val=1, arith_type_sgadvanced=, arith_type=Unsigned, n_bits=ceil(log(delay_len-bram_latency)/log(2)), bin_pt=0, load_pin_sgadvanced=, load_pin=off, rst_sgadvanced=, rst=off, en_sgadvanced=, en=off, explicit_period_sgadvanced=, explicit_period=on, period=1, dbl_ovrd_sgadvanced=, dbl_ovrd=off, use_behavioral_HDL_sgadvanced=, use_behavioral_HDL=off, implementation_sgadvanced=, implementation=Fabric, xl_use_area_sgadvanced=, xl_use_area=off, xl_area=[0, 0, 0, 0, 0, 0, 0], use_rpm=off, xlcconfig=, has_advanced_control=0, sggui_pos=-1,-1,-1,-1, block_type=counter, block_version=9.1.01, sg_icon_stat=40,40,0,1,white,blue,0,4b061529,right,,[ ],[ ], sg_mask_display=|, sg_list_contents=, sg_blockgui_xml=}
      mask sg_mask_display=|
      | fprintf('','COMMENT: begin icon graphics');
      | patch([0 40 40 0 0 ],[0 0 40 40 0 ],[0.77 0.82 0.91 ]);
      | plot([0 40 40 0 0 ],[0 0 40 40 0 ]);
      | patch([8.875 16.1 21.1 26.1 31.1 21.1 13.875 8.875 ],[25.55 25.55 30.55 25.55 30.55 30.55 30.55 25.55 ],[1 1 1 ]);
      | patch([13.875 21.1 16.1 8.875 13.875 ],[20.55 20.55 25.55 25.55 20.55 ],[0.931 0.946 0.973 ]);
      | patch([8.875 16.1 21.1 13.875 8.875 ],[15.55 15.55 20.55 20.55 15.55 ],[1 1 1 ]);
      | patch([13.875 31.1 26.1 21.1 16.1 8.875 13.875 ],[10.55 10.55 15.55 10.55 15.55 15.55 10.55 ],[0.931 0.946 0.973 ]);
      | fprintf('','COMMENT: end icon graphics');
      | fprintf('','COMMENT: begin icon text');
      |
      | color('black');disp('{\fontsize{14}\bf\lceil++\rceil}','texmode','on');
      | fprintf('','COMMENT: end icon text');
      mask prompts: infoedit ""; cnt_type_sgadvanced ""; cnt_type "Counter type"; cnt_to "Count to value"; operation_sgadvanced ""; operation "Count direction"; start_count "Initial value"; cnt_by_val "Step"; arith_type_sgadvanced ""; arith_type "Output type"; n_bits "Number of bits"; bin_pt "Binary point"; load_pin_sgadvanced ""; load_pin "Provide load port"; rst_sgadvanced ""; rst "Provide synchronous reset port"; en_sgadvanced ""; en "Provide enable port"; explicit_period_sgadvanced ""; explicit_period "Sample period source"; period "Explicit period"; dbl_ovrd_sgadvanced ""; dbl_ovrd "Override with doubles"; use_behavioral_HDL_sgadvanced ""; use_behavioral_HDL "Use behavioral HDL (otherwise use core)"; implementation_sgadvanced ""; implementation "Implement using"; xl_use_area_sgadvanced ""; xl_use_area "Define FPGA area for resource estimation"; xl_area "FPGA area [slices, FFs, BRAMs, LUTs, IOBs, emb. mults, TBUFs]"; use_rpm ""; xlcconfig ""; has_advanced_control ""; sggui_pos ""; block_type ""; block_version ""; sg_icon_stat ""; sg_mask_display ""; sg_list_contents ""; sg_blockgui_xml ""
      mask help: Hardware notes: Free running counters are the least expensive in hardware. A count limited counter is implemented by combining a counter with a comparator.
      mask init: same as monroe_library/counter_limited_fast/Counter1
      settings: CopyFcn=xlBlockMoveCallback(gcbh);  DeleteFcn=xlDestroyGui(gcbh);  ModelCloseFcn=xlDestroyGui(gcbh);  PreSaveFcn=xlBlockPreSaveCallback(gcbh);  PostSaveFcn=xlBlockPostSaveCallback(gcbh);  DestroyFcn=xlDestroyGui(gcbh);  OpenFcn=xlOpenGui(gcbh, 'counter_gui.xml', @counterenablement, -1)  CloseFcn=xlDestroyGui(gcbh);  MoveFcn=xlBlockMoveCallback(gcbh);
      mask Help: eval('');xlDoc('-book','sysgen','-topic','Counter');
      mask TypeOptions cnt_type: Free Running | Count Limited
      mask TypeOptions operation: Up | Down | Up/Down
      mask TypeOptions arith_type: Signed  (2's comp) | Unsigned
      mask TypeOptions explicit_period: on | off
      mask TypeOptions implementation: Fabric | DSP48
      mask Display:
      | fprintf('','COMMENT: begin icon graphics');
      | patch([0 40 40 0 0 ],[0 0 40 40 0 ],[0.77 0.82 0.91 ]);
      | plot([0 40 40 0 0 ],[0 0 40 40 0 ]);
      | patch([8.875 16.1 21.1 26.1 31.1 21.1 13.875 8.875 ],[25.55 25.55 30.55 25.55 30.55 30.55 30.55 25.55 ],[1 1 1 ]);
      | patch([13.875 21.1 16.1 8.875 13.875 ],[20.55 20.55 25.55 25.55 20.55 ],[0.931 0.946 0.973 ]);
      | patch([8.875 16.1 21.1 13.875 8.875 ],[15.55 15.55 20.55 20.55 15.55 ],[1 1 1 ]);
      | patch([13.875 31.1 26.1 21.1 16.1 8.875 13.875 ],[10.55 10.55 15.55 10.55 15.55 15.55 10.55 ],[0.931 0.946 0.973 ]);
      | fprintf('','COMMENT: end icon graphics');
      | fprintf('','COMMENT: begin icon text');
      | 
      | color('black');disp('{\fontsize{14}\bf\lceil++\rceil}','texmode','on');
      | fprintf('','COMMENT: end icon text');
  Single Port RAM : xbsIndex_r4/Single Port RAM  depth=2^ceil(log(2*(delay_len-bram_latency))/log(2))  initVector=0  distributed_mem=Distributed memory  write_mode=Read Before Write  rst=off  init_reg=0  en=off  latency=bram_latency  dbl_ovrd=off  optimize=Area  use_rpm=on  block_type=spram
  Single Port RAM1 : S-Function  LoadFcn=xlBlockLoadCallback(gcbh);  FunctionName=sysgen  Parameters=ptable_  EnableBusSupport=off  mask(Xilinx Single Port Random Access Memory Block){depth=2^ceil(log(2*(delay_len-bram_latency))/log(2)), initVector=0, distributed_mem_sgadvanced=, distributed_mem=Distributed memory, write_mode_sgadvanced=, write_mode=Read Before Write, rst_sgadvanced=, rst=off, init_reg=0, en_sgadvanced=, en=off, latency=bram_latency, dbl_ovrd_sgadvanced=, dbl_ovrd=off, optimize_sgadvanced=, optimize=Area, use_rpm_sgadvanced=, use_rpm=on, xl_use_area_sgadvanced=, xl_use_area=off, xl_area=[0,0,0,0,0,0,0], has_advanced_control=0, sggui_pos=-1,-1,-1,-1, block_type=spram, block_version=, sg_icon_stat=70,106,3,1,white,blue,0,0b4315b4,right,,[ ],[ ], sg_mask_display=|, sg_list_contents=, sg_blockgui_xml=}
      mask sg_mask_display=|
      | fprintf('','COMMENT: begin icon graphics');
      | patch([0 70 70 0 0 ],[0 0 106 106 0 ],[0.77 0.82 0.91 ]);
      | plot([0 70 70 0 0 ],[0 0 106 106 0 ]);
      | patch([12.75 27.2 37.2 47.2 57.2 37.2 22.75 12.75 ],[64.1 64.1 74.1 64.1 74.1 74.1 74.1 64.1 ],[1 1 1 ]);
      | patch([22.75 37.2 27.2 12.75 22.75 ],[54.1 54.1 64.1 64.1 54.1 ],[0.931 0.946 0.973 ]);
      | patch([12.75 27.2 37.2 22.75 12.75 ],[44.1 44.1 54.1 54.1 44.1 ],[1 1 1 ]);
      | patch([22.75 57.2 47.2 37.2 27.2 12.75 22.75 ],[34.1 34.1 44.1 34.1 44.1 44.1 34.1 ],[0.931 0.946 0.973 ]);
      | fprintf('','COMMENT: end icon graphics');
      | fprintf('','COMMENT: begin icon text');
      | color('black');port_label('input',1,'addr');
      | color('black');port_label('input',2,'data');
      | color('black');port_label('input',3,'we');
      |
      | color('black');disp('z^{-3}','texmode','on');
      | fprintf('','COMMENT: end icon text');
      mask prompts: initVector "Initial value vector"; distributed_mem_sgadvanced ""; distributed_mem "Memory Type"; write_mode_sgadvanced ""; write_mode "Write Mode"; rst_sgadvanced ""; rst "Provide reset port for output register"; init_reg "Initial value for output register"; en_sgadvanced ""; en "Provide enable port"; dbl_ovrd_sgadvanced ""; dbl_ovrd "Override with doubles"; optimize_sgadvanced ""; optimize "Optimize for"; use_rpm_sgadvanced ""; use_rpm "Use pre-defined core placement information"; xl_use_area_sgadvanced ""; xl_use_area "Define FPGA area for resource estimation"; xl_area "FPGA area [slices, FFs, BRAMs, LUTs, IOBs, emb. mults, TBUFs]"; has_advanced_control ""; sggui_pos ""; block_type ""; block_version ""; sg_icon_stat ""; sg_mask_display ""; sg_list_contents ""; sg_blockgui_xml ""
      mask help: Xilinx Single Port Random Access Memory
      mask init:
      | try
      |   tmp_gcb = gcb;
      |   tmp_gcbh = gcbh;
      |   if (strcmp('SysGenIndex',get_param(bdroot(tmp_gcbh),'tag')) && ~isempty(regexp(bdroot(tmp_gcb), '^xbs', 'once')))
      |     return;
      |   end;
      |   xlMungeMaskParams;
      |   block_config = 'sysgen_blockset:SPRAM_config';
      | 
      |   block_type='spram';
      | 
      |   serialized_declarations = '{''depth''=>''Int'',''distributed_mem''=>''Int'',''en''=>''Int'',''initVector''=>''DoubleVector'',''init_reg''=>''Double'',''latency''=>''Int'',''optimize''=>''Int'',''rst''=>''Int'',''use_rpm''=>''Int'',''write_mode''=>''Int'',''block_type''=>''String''}';
      |   xlspram_init();
      |   ptable_ = xlblockprep(get_param(tmp_gcb, 'MaskWSVariables'));
      |   try
      |     xlBlockMoveCallback(tmp_gcbh);
      |   catch 
      |      clear global xl_updateicon_recursion_guard;
      |   end;
      | catch
      |   global dbgsysgen;
      |   if(~isempty(dbgsysgen) && dbgsysgen)
      |     e = regexprep(lasterr, '\n', '\nError: ');
      |     disp(['Error: While running MaskInit code on block ' tmp_gcb ': ' e]);
      |     error(e);
      |   end
      | end
      settings: CopyFcn=xlBlockMoveCallback(gcbh);  DeleteFcn=xlDestroyGui(gcbh);  ModelCloseFcn=xlDestroyGui(gcbh);  PreSaveFcn=xlBlockPreSaveCallback(gcbh);  PostSaveFcn=xlBlockPostSaveCallback(gcbh);  DestroyFcn=xlDestroyGui(gcbh);  OpenFcn=xlOpenGui(gcbh, 'spram_gui.xml', @spramenablement, -1)  CloseFcn=xlDestroyGui(gcbh);  MoveFcn=xlBlockMoveCallback(gcbh);
      mask Help: eval('');xlDoc('-book','sysgen','-topic','Single_Port_RAM');
      mask TypeOptions distributed_mem: Distributed memory | Block RAM
      mask TypeOptions write_mode: Read After Write | Read Before Write | No Read On Write
      mask TypeOptions optimize: Area | Speed
      mask Display:
      | fprintf('','COMMENT: begin icon graphics');
      | patch([0 70 70 0 0 ],[0 0 106 106 0 ],[0.77 0.82 0.91 ]);
      | plot([0 70 70 0 0 ],[0 0 106 106 0 ]);
      | patch([12.75 27.2 37.2 47.2 57.2 37.2 22.75 12.75 ],[64.1 64.1 74.1 64.1 74.1 74.1 74.1 64.1 ],[1 1 1 ]);
      | patch([22.75 37.2 27.2 12.75 22.75 ],[54.1 54.1 64.1 64.1 54.1 ],[0.931 0.946 0.973 ]);
      | patch([12.75 27.2 37.2 22.75 12.75 ],[44.1 44.1 54.1 54.1 44.1 ],[1 1 1 ]);
      | patch([22.75 57.2 47.2 37.2 27.2 12.75 22.75 ],[34.1 34.1 44.1 34.1 44.1 44.1 34.1 ],[0.931 0.946 0.973 ]);
      | fprintf('','COMMENT: end icon graphics');
      | fprintf('','COMMENT: begin icon text');
      | color('black');port_label('input',1,'addr');
      | color('black');port_label('input',2,'data');
      | color('black');port_label('input',3,'we');
      | 
      | color('black');disp('z^{-3}','texmode','on');
      | fprintf('','COMMENT: end icon text');
  outA : Outport
  outB : Outport  Port=2
  wires:
  Constant3/1 -> Concat1/1
  Concat/1 -> Single Port RAM/1
  Constant1/1 -> Concat/1
  Counter/1 -> Concat1/2, Concat/2
  Constant2/1 -> Single Port RAM/3, Single Port RAM1/3
  inB/1 -> Single Port RAM1/2
  inA/1 -> Single Port RAM/2
  Single Port RAM1/1 -> outB/1
  Single Port RAM/1 -> outA/1
  Concat1/1 -> Single Port RAM1/1
